simulink model "PROJECT_LATEST2"  (R2023a)
settings: Solver=VariableStepAuto  StartTime=0.0  StopTime=0.5  RelTol=1e-3
libraries: spsDiodeLib x4, spsIGBTDiodeLib x4, spsSeriesRLCBranchLib x4, spsVoltageMeasurementLib x4, spsCurrentMeasurementLib x3, spsDCVoltageSourceLib x1, spsLinearTransformerLib x1, spsMeanLib x1, sps_lib x1
settings Model: Creator=bpven  LastModifiedBy=yadur
settings SolverCC: ZeroCrossAlgorithm=Adaptive
settings DataIOCC: SaveFormat=StructureWithTime
settings DebuggingCC: MaskedZcDiagnostic=none  IgnoredZcDiagnostic=none

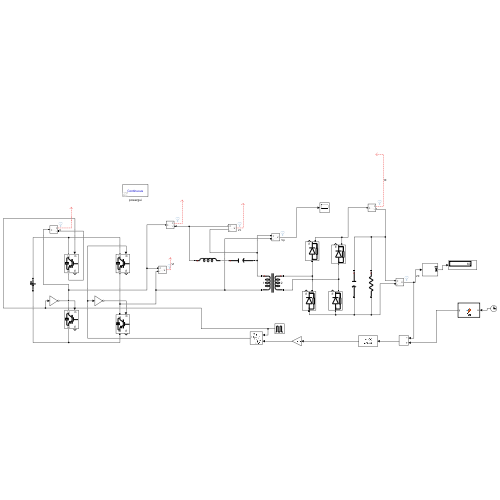
[thumbnail: Simulink's stored preview of the top-level diagram]
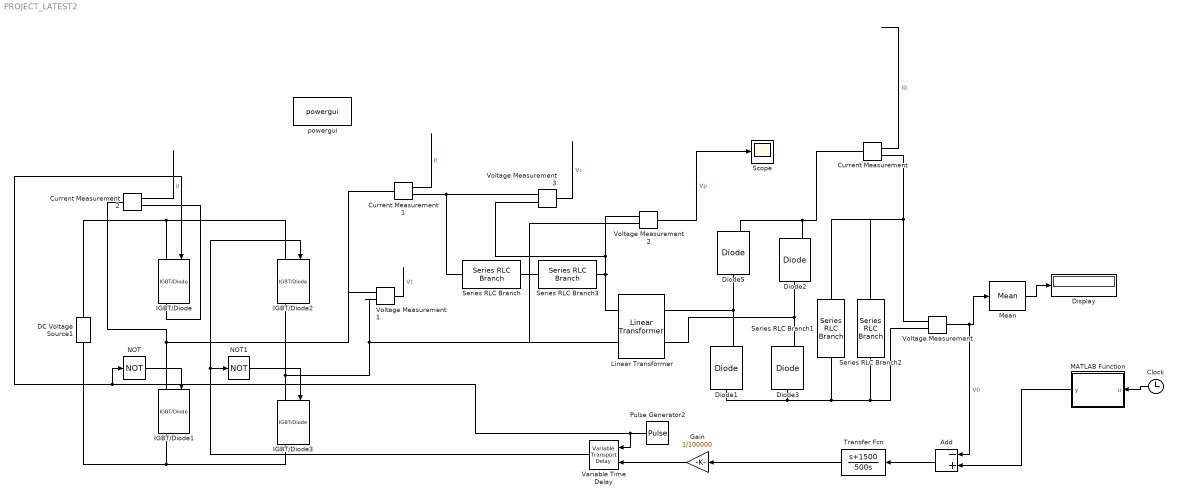
== system PROJECT_LATEST2 ==
  Add : Sum  Inputs=-+
  Clock : Clock
  Current Measurement : spsCurrentMeasurementLib/Current Measurement  PhasorSimulation=off  OutputType=Complex  PSBequivalent=0
  Current Measurement1 : spsCurrentMeasurementLib/Current Measurement  PhasorSimulation=off  OutputType=Complex  PSBequivalent=0
  Current Measurement2 : spsCurrentMeasurementLib/Current Measurement  PhasorSimulation=off  OutputType=Complex  PSBequivalent=0
  DC Voltage Source1 : spsDCVoltageSourceLib/DC Voltage Source  Amplitude=400  Measurements=None
  Diode{1..3,5} (4 alike) : spsDiodeLib/Diode  Ron=0.001  Lon=0  Vf=0  IC=0  UseSnubber=0  Rs=500  Cs=250e-9  Measurements=on
  Display : Display
  Gain : Gain  Gain=1/100000
  IGBT/Diode{,1..3} (4 alike) : spsIGBTDiodeLib/IGBT//Diode  Ron=1e-3  Rs=1e5  Cs=inf  Measurements=on
  Linear Transformer : spsLinearTransformerLib/Linear Transformer  UNITS=SI  NominalPower=[ 1e3 100000 ]  winding1=[1000 0 0]  winding2=[400 0 0]  ThreeWindings=off  winding3=[3.15e+05 99225 0.63169]  RmLm=[1e6 2286.61]  Measurements=All voltages and currents  DataType=on
  MATLAB Function : MATLAB Function  TreatAsAtomicUnit=on
  Mean : spsMeanLib/Mean  Freq=50  Vinit=0  Ts=0
  NOT : Logic  Operator=NOT  IconShape=distinctive  AllPortsSameDT=off  OutDataTypeStr=boolean
  NOT1 : Logic  Operator=NOT  IconShape=distinctive  AllPortsSameDT=off  OutDataTypeStr=boolean
  Pulse Generator2 : DiscretePulseGenerator  PulseType=Time based  Period=1e-5  PulseWidth=50
  Scope : Scope
  Series RLC Branch : spsSeriesRLCBranchLib/Series RLC Branch  LConnTagsString=__new0  RConnTagsString=__new0  BranchType=L  Resistance=1  Inductance=379.4e-6  SetiL0=off  InitialCurrent=0  Capacitance=1e-8  Setx0=off  InitialVoltage=0  Measurements=None
  Series RLC Branch1 : spsSeriesRLCBranchLib/Series RLC Branch  LConnTagsString=__new0  RConnTagsString=__new0  BranchType=C  Resistance=1.152  Inductance=1e-3  SetiL0=off  InitialCurrent=0  Capacitance=100e-6  Setx0=off  InitialVoltage=0  Measurements=None
  Series RLC Branch2 : spsSeriesRLCBranchLib/Series RLC Branch  LConnTagsString=__new0  RConnTagsString=__new0  BranchType=R  Resistance=2.304  Inductance=1e-3  SetiL0=off  InitialCurrent=0  Capacitance=1e-6  Setx0=off  InitialVoltage=0  Measurements=None
  Series RLC Branch3 : spsSeriesRLCBranchLib/Series RLC Branch  LConnTagsString=__new0  RConnTagsString=__new0  BranchType=C  Resistance=1.152  Inductance=1e-3  SetiL0=off  InitialCurrent=0  Capacitance=6.676e-9  Setx0=off  InitialVoltage=0  Measurements=None
  Transfer Fcn : TransferFcn  Numerator=[1 1500]  Denominator=[500 0]
  Variable Time Delay : VariableTransportDelay  MaximumDelay=10
  Voltage Measurement{,1..3} (4 alike) : spsVoltageMeasurementLib/Voltage Measurement  PhasorSimulation=off  OutputType=Complex  PSBequivalent=0
  powergui : sps_lib/powergui  Priority=1  SimulationMode=Continuous  SampleTime=50e-6  frequency=60  Iterations=50  frequencyindice=0  Pbase=100e6  ErrMax=1e-4  UnitsV=kV  UnitsW=MW  buscounter=0  FunctionMessages=off  echomessages=off  EnableUseOfTLC=off  CurrentSourceSwitches=off  DisableSnubberDevices=off  DisableRonSwitches=off  DisableVfSwitches=off  DisplayEquations=off  AutomaticDiscreteSolvers=off  SolverType=Tustin/Backward Euler (TBE)  Interpol=off  ExternalGateDelay=off  methode=off  Ts=100  x0status=blocks  SPID=on  SwTol=0  HookPort=off  NonlinearTolerance=1e-4  nMaxIteration=100  ContinueOnMaxIteration=off  RestoreLinks=warning  ResistiveCurrentMeasurement=off  Frange=[0:2:500]  Ylog=off  Xlog=on  ShowGrid=off  save=off  variable=ZData  structure=0  ZoomFFT=off  StartTime=0.0  cycles=1  DisplayStyle=1  fundamental=60  FreqAxis=off  MaxFrequency=1000  frequencyindicesteady=1  RmsSteady=1  display=off
  wires:
  NOT/1 -> IGBT/Diode1/1
  Voltage Measurement1/1 -> ?  "Vt"
  Voltage Measurement/1 -> Add/1, Mean/1  "V0"
  NOT1/1 -> IGBT/Diode3/1
  Mean/1 -> Display/1
  Pulse Generator2/1 -> Variable Time Delay/1, NOT/1, IGBT/Diode/1
  Voltage Measurement2/1 -> Scope/1  "Vp"
  Current Measurement/1 -> ?  "I0"
  Current Measurement1/1 -> ?  "Il"
  Voltage Measurement3/1 -> ?  "Vc"
  Gain/1 -> Variable Time Delay/2
  Add/1 -> Transfer Fcn/1
  Clock/1 -> MATLAB Function/1(u)
  Variable Time Delay/1 -> IGBT/Diode2/1, NOT1/1
  Transfer Fcn/1 -> Gain/1
  MATLAB Function/1(y) -> Add/2
  Current Measurement2/1 -> ?  "Il"
  connections:
  Voltage Measurement1/LConn2 -- Linear Transformer/LConn2 -- Voltage Measurement2/LConn2 -- IGBT/Diode3/LConn1 -- IGBT/Diode2/RConn1
  DC Voltage Source1/RConn1 -- IGBT/Diode/LConn1 -- IGBT/Diode2/LConn1
  IGBT/Diode1/LConn1 -- Voltage Measurement1/LConn1 -- Current Measurement1/LConn1 -- Current Measurement2/LConn1
  DC Voltage Source1/LConn1 -- IGBT/Diode1/RConn1 -- IGBT/Diode3/RConn1
  Voltage Measurement2/LConn1 -- Linear Transformer/LConn1 -- Series RLC Branch3/RConn1 -- Voltage Measurement3/LConn2
  Linear Transformer/RConn1 -- Diode5/LConn1 -- Diode1/RConn1
  Linear Transformer/RConn2 -- Diode2/LConn1 -- Diode3/RConn1
  Voltage Measurement/LConn1 -- Series RLC Branch1/LConn1 -- Series RLC Branch2/LConn1 -- Current Measurement/RConn1
  Voltage Measurement/LConn2 -- Series RLC Branch2/RConn1 -- Series RLC Branch1/RConn1 -- Diode3/LConn1 -- Diode1/LConn1
  Diode5/RConn1 -- Current Measurement/LConn1 -- Diode2/RConn1
  Current Measurement1/RConn1 -- Series RLC Branch/LConn1 -- Voltage Measurement3/LConn1
  Series RLC Branch3/LConn1 -- Series RLC Branch/RConn1
  Current Measurement2/RConn1 -- IGBT/Diode/RConn1

== matlab function PROJECT_LATEST2/MATLAB Function ==
  data: u input; y output
function y = fcn(u)

if(u<0.2)
   y = 48;
else
    y=60;
end 
end
